simulink model "paralelo3usinas"  (Simulink 7.5)
settings: Solver=ode45  StartTime=0.0  StopTime=500  MaxStep=100  RelTol=1e-3
values from neighbouring files (symbols this model uses):
  B1 = 0.6    [princ_paralelo3usinas.m]
  B2 = 0.6    [princ_paralelo3usinas.m]
  C1 = 0.6    [princ_paralelo3usinas.m]
  C2 = 0.6    [princ_paralelo3usinas.m]
  DPD_pu1 = DPD/PB    (= 0.042296)    [sistema1.m]
  DPD_pu2 = DPD/PB    (= 0.070494)    [sistema2.m]
  DPD_pu3 = DPD/PB    (= 0.11279)    [sistema3.m]
  Gest = 0.0586    [princ_paralelo3usinas.m]
  Gsae = 0.1250    (= 0.125)    [princ_paralelo3usinas.m]
  K12 = cos(teta12)/X12    [princ_paralelo3usinas.m]
  K1_12 = sin (teta12)/X12    [princ_paralelo3usinas.m]
  K1_23 = sin (teta23)/X23    [princ_paralelo3usinas.m]
  K23 = cos(teta23)/X23    [princ_paralelo3usinas.m]
  K2_12 = sin(teta12)/X12    [princ_paralelo3usinas.m]
  Kd1 = 0.0586    [princ_paralelo3usinas.m]
  Kd2 = 3.2410    (= 3.241)    [princ_paralelo3usinas.m]
  Kd3 = 0.2826    [princ_paralelo3usinas.m]
  Ki1 = 0.0092    [princ_paralelo3usinas.m]
  Ki2 = 0.0541    [princ_paralelo3usinas.m]
  Kp1 = -0.0242    [princ_paralelo3usinas.m]
  Kp2 = -0.2928    [princ_paralelo3usinas.m]
  Kp3 = 0.3558    [princ_paralelo3usinas.m]
  Kps1 = 1/D_pu    (= 88.922039025)    [sistema1.m]
  Kps2 = 1/D_pu    (= 10.0350855099)    [sistema2.m]
  Kps3 = 1/D_pu    (= 15.8041808295)    [sistema3.m]
  PD_pu1 = PD/PB    (= 1.13594)    [sistema1.m]
  PD_pu2 = PD/PB    (= 1.893234)    [sistema2.m]
  REG_pu1 = REG/PB    (= 1.64172103535)    [sistema1.m]
  REG_pu2 = REG/PB    (= 1.31995425045)    [sistema2.m]
  REG_pu3 = REG/PB    (= 0.108094752772)    [sistema3.m]
  T1 = 0.1013    [princ_paralelo3usinas.m]
  T2 = 0.1238    [princ_paralelo3usinas.m]
  Ta = 0.4401    [princ_paralelo3usinas.m]
  Tb = 0.08    [princ_paralelo3usinas.m]
  Test = 0.0223    [princ_paralelo3usinas.m]
  TG1 = 0.6419    [sistema1.m]
  TG2 = 0.6002    [sistema2.m]
  TG3 = 0.4505    [sistema3.m]
  Tps1 = 2*H_pu/(D_pu*f0)    (= 48.2838817126)    [sistema1.m]
  Tps2 = 2*H_pu/(D_pu*f0)    (= 8.70581433357)    [sistema2.m]
  Tps3 = 2*H_pu/(D_pu*f0)    (= 1.06634811782)    [sistema3.m]
  Tt1 = 5.7257    [princ_paralelo3usinas.m]
  Tt2 = 1.0740    (= 1.074)    [princ_paralelo3usinas.m]
  Tt3 = 1.0552    [princ_paralelo3usinas.m]
  TW1 = 1.0882    [sistema1.m]
  TW2 = 1.2650    (= 1.265)    [sistema2.m]
  TW3 = 1.3430    (= 1.343)    [sistema3.m]
settings Model: Creator=Edimar  LastModifiedBy=Laís  ExtModeTrigMode=oneshot  ExtModeArmWhenConnect=off
settings DataIOCC: LimitDataPoints=off
settings OptimizationCC: BooleanDataType=off
settings DebuggingCC: SaveWithParameterizedLinksMsg=none  SignalResolutionControl=TryResolveAllWithWarning  SolverPrmCheckMsg=none  MultiTaskDSMMsg=warning  MultiTaskCondExecSysMsg=none  StrictBusMsg=None
settings HardwareCC: TargetUnknown=on
settings RTWCC: IncludeERTFirstTime=on

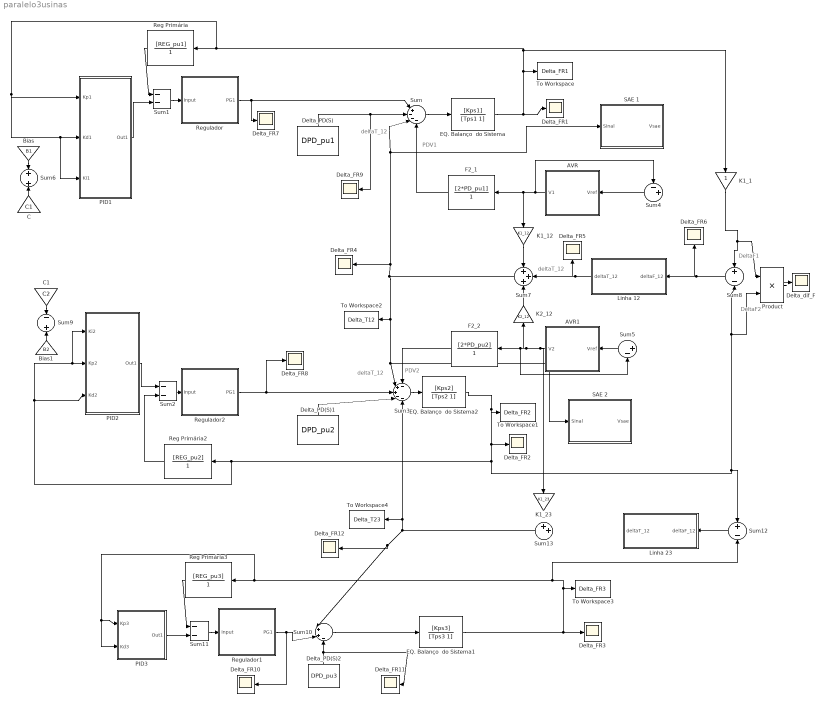
== system paralelo3usinas ==
  note: PDV1
  note: PDV2
  note: DeltaF1
  note: DeltaF2
  note: deltaT_12
  note: deltaT_12
  note: deltaT_12
  AVR : Subsystem
  AVR1 : Subsystem
  Bias : Gain  Gain=B1  ParameterDataType=fixdt(1, 16)  ParameterScaling=2^0  OutDataType=fixdt(1, 16)  OutScaling=2^0
  Bias1 : Gain  Gain=B2  ParameterDataType=fixdt(1, 16)  ParameterScaling=2^0  OutDataType=fixdt(1, 16)  OutScaling=2^0
  C : Gain  Gain=C1  ParameterDataType=fixdt(1, 16)  ParameterScaling=2^0  OutDataType=fixdt(1, 16)  OutScaling=2^0
  C1 : Gain  Gain=C2  ParameterDataType=fixdt(1, 16)  ParameterScaling=2^0  OutDataType=fixdt(1, 16)  OutScaling=2^0
  Delta_FR{1..12} (12 alike) : Scope
      Delta_FR1 settings: Description=tetetet  TimeRange=1000  YMin=-4  YMax=3
      Delta_FR10 settings: Description=tetetet  TimeRange=1000  YMin=-4  YMax=3  SaveName=ScopeData11  MaxDataPoints=5000000
      Delta_FR11 settings: Description=tetetet  TimeRange=1000  YMin=-4  YMax=3  SaveName=ScopeData12  MaxDataPoints=5000000
      Delta_FR12 settings: Description=tetetet  TimeRange=1000  YMin=-4  YMax=3  SaveName=ScopeData13  MaxDataPoints=5000000
      Delta_FR2 settings: Description=tetetet  TimeRange=1000  YMin=-4  YMax=3  SaveName=ScopeData3
      Delta_FR3 settings: Description=tetetet  TimeRange=1000  YMin=-4  YMax=3  SaveName=ScopeData9
      Delta_FR4 settings: Description=tetetet  TimeRange=1000  YMin=-4  YMax=3  SaveName=ScopeData8  MaxDataPoints=5000000
      Delta_FR5 settings: Description=tetetet  TimeRange=1000  YMin=-4  YMax=3  SaveName=ScopeData4
      Delta_FR6 settings: Description=tetetet  TimeRange=1000  YMin=-4  YMax=3  SaveName=ScopeData5
      Delta_FR7 settings: Description=tetetet  TimeRange=1000  YMin=-4  YMax=3  SaveName=ScopeData6  MaxDataPoints=5000000
      Delta_FR8 settings: Description=tetetet  TimeRange=1000  YMin=-4  YMax=3  SaveName=ScopeData7
      Delta_FR9 settings: Description=tetetet  TimeRange=1000  YMin=-4  YMax=3  SaveName=ScopeData10  MaxDataPoints=5000000
  Delta_PD(S) : Constant  Value=DPD_pu1
  Delta_PD(S)1 : Constant  Value=DPD_pu2
  Delta_PD(S)2 : Constant  Value=DPD_pu3
  Delta_dif_F : Scope
      settings: Description=tetetet  TimeRange=1000  YMin=-4  YMax=3
  EQ. Balanço  do Sistema : TransferFcn  Numerator=[Kps1]  Denominator=[Tps1 1]
  EQ. Balanço  do Sistema1 : TransferFcn  Numerator=[Kps3]  Denominator=[Tps3 1]
  EQ. Balanço  do Sistema2 : TransferFcn  Numerator=[Kps2]  Denominator=[Tps2 1]
  F2_1 : TransferFcn  Numerator=[2*PD_pu1]  Denominator=[0 1]
  F2_2 : TransferFcn  Numerator=[2*PD_pu2]  Denominator=[0 1]
  K1_1 : Gain  ParameterDataType=fixdt(1, 16)  ParameterScaling=2^0  OutDataType=fixdt(1, 16)  OutScaling=2^0
  K1_12 : Gain  Gain=K1_12  ParameterDataType=fixdt(1, 16)  ParameterScaling=2^0  OutDataType=fixdt(1, 16)  OutScaling=2^0
  K1_23 : Gain  Gain=K1_23  ParameterDataType=fixdt(1, 16)  ParameterScaling=2^0  OutDataType=fixdt(1, 16)  OutScaling=2^0
  K2_12 : Gain  Gain=K2_12  ParameterDataType=fixdt(1, 16)  ParameterScaling=2^0  OutDataType=fixdt(1, 16)  OutScaling=2^0
  Linha 12 : Subsystem
  Linha 23 : Subsystem
  PID1 : Subsystem
  PID2 : Subsystem
  PID3 : Subsystem
  Product : Product  OutDataType=fixdt(1, 16)  OutScaling=2^0  RndMeth=Zero
  Reg Primária : TransferFcn  Numerator=[REG_pu1]  Denominator=[0 1]
  Reg Primária2 : TransferFcn  Numerator=[REG_pu2]  Denominator=[0 1]
  Reg Primária3 : TransferFcn  Numerator=[REG_pu3]  Denominator=[0 1]
  Regulador : Subsystem
  Regulador1 : Subsystem
  Regulador2 : Subsystem
  SAE 1 : Subsystem
  SAE 2 : Subsystem
  Sum : Sum  Inputs=|+---  SaturateOnIntegerOverflow=on  InputSameDT=on  OutDataTypeStr=Inherit: Same as first input
  Sum1 : Sum  Inputs=--  SaturateOnIntegerOverflow=on  InputSameDT=on  OutDataTypeStr=Inherit: Same as first input
  Sum10 : Sum  Inputs=|++-  SaturateOnIntegerOverflow=on  InputSameDT=on  OutDataTypeStr=Inherit: Same as first input
  Sum11 : Sum  Inputs=--  SaturateOnIntegerOverflow=on  InputSameDT=on  OutDataTypeStr=Inherit: Same as first input
  Sum12 : Sum  Inputs=+|-  OutDataType=fixdt(1, 16)  OutScaling=2^0
  Sum13 : Sum  Inputs=++|  SaturateOnIntegerOverflow=on  InputSameDT=on  OutDataTypeStr=Inherit: Same as first input
  Sum2 : Sum  Inputs=--  SaturateOnIntegerOverflow=on  InputSameDT=on  OutDataTypeStr=Inherit: Same as first input
  Sum3 : Sum  Inputs=-++--  SaturateOnIntegerOverflow=on  InputSameDT=on  OutDataTypeStr=Inherit: Same as first input
  Sum4 : Sum  Inputs=-+|  SaturateOnIntegerOverflow=on  InputSameDT=on  OutDataTypeStr=Inherit: Same as first input
  Sum5 : Sum  Inputs=|+-  SaturateOnIntegerOverflow=on  InputSameDT=on  OutDataTypeStr=Inherit: Same as first input
  Sum6 : Sum  Inputs=+|+  SaturateOnIntegerOverflow=on  InputSameDT=on  OutDataTypeStr=Inherit: Same as first input
  Sum7 : Sum  Inputs=+++  SaturateOnIntegerOverflow=on  InputSameDT=on  OutDataTypeStr=Inherit: Same as first input
  Sum8 : Sum  Inputs=+|-  OutDataType=fixdt(1, 16)  OutScaling=2^0
  Sum9 : Sum  Inputs=-|+  SaturateOnIntegerOverflow=on  InputSameDT=on  OutDataTypeStr=Inherit: Same as first input
  To Workspace : ToWorkspace  VariableName=Delta_FR1  SampleTime=-1  SaveFormat=Array
  To Workspace1 : ToWorkspace  VariableName=Delta_FR2  SampleTime=-1  SaveFormat=Array
  To Workspace2 : ToWorkspace  VariableName=Delta_T12  SampleTime=-1  SaveFormat=Array
  To Workspace3 : ToWorkspace  VariableName=Delta_FR3  SampleTime=-1  SaveFormat=Array
  To Workspace4 : ToWorkspace  VariableName=Delta_T23  SampleTime=-1  SaveFormat=Array
  wires:
  Delta_PD(S)/1 -> Sum/2, Delta_FR9/1
  EQ. Balanço  do Sistema/1 -> Delta_FR1/1, To Workspace/1, Reg Primária/1, PID1/1(Kp1), PID1/2(Kd1), PID1/3(Ki1), K1_1/1
  Sum/1 -> EQ. Balanço  do Sistema/1
  AVR/1(V1) -> Sum4/1, F2_1/1, K1_12/1
  Sum4/1 -> AVR/1(Vref)
  Sum3/1 -> EQ. Balanço  do Sistema2/1
  EQ. Balanço  do Sistema2/1 -> To Workspace1/1, Delta_FR2/1, Reg Primária2/1, PID2/3(Kd2), PID2/2(Kp2), PID2/1(Ki2), Product/2, Sum8/2, Sum12/1
  Sum5/1 -> AVR1/1(Vref)
  AVR1/1(V2) -> Sum5/2, F2_2/1, K2_12/1, K1_23/1
  F2_2/1 -> Sum3/1
  Delta_PD(S)1/1 -> Sum3/4
  F2_1/1 -> Sum/4
  PID1/1(Out1) -> Sum1/2
  Reg Primária/1 -> Sum1/1
  Sum1/1 -> Regulador/1(Input)
  Regulador/1(PG1) -> Sum/1, Delta_FR7/1
  Sum2/1 -> Regulador2/1(Input)
  PID2/1(Out1) -> Sum2/1
  Reg Primária2/1 -> Sum2/2
  Regulador2/1(PG1) -> Sum3/3, Delta_FR8/1
  Linha 12/1(deltaT_12) -> Sum7/2, Delta_FR5/1
  Product/1 -> Delta_dif_F/1
  Sum8/1 -> Linha 12/1(deltaF_12), Delta_FR6/1
  K1_1/1 -> Product/1, Sum8/1
  Sum7/1 -> Delta_FR4/1, Sum/3, SAE 1/1(Sinal), To Workspace2/1, Sum3/2, SAE 2/1(Sinal)
  K2_12/1 -> Sum7/3
  K1_12/1 -> Sum7/1
  Bias/1 -> Sum6/1
  C/1 -> Sum6/2
  C1/1 -> Sum9/1
  Bias1/1 -> Sum9/2
  EQ. Balanço  do Sistema1/1 -> Delta_FR3/1, To Workspace3/1, Reg Primária3/1, PID3/1(Kp3), PID3/2(Kd3), Sum12/2
  Sum10/1 -> EQ. Balanço  do Sistema1/1
  PID3/1(Out1) -> Sum11/2
  Reg Primária3/1 -> Sum11/1
  Sum11/1 -> Regulador1/1(Input)
  Sum12/1 -> Linha 23/1(deltaF_12)
  Regulador1/1(PG1) -> Sum10/2, Delta_FR10/1
  Delta_PD(S)2/1 -> Sum10/3, Delta_FR11/1
  Sum13/1 -> Sum3/5, To Workspace4/1, Sum10/1, Delta_FR12/1

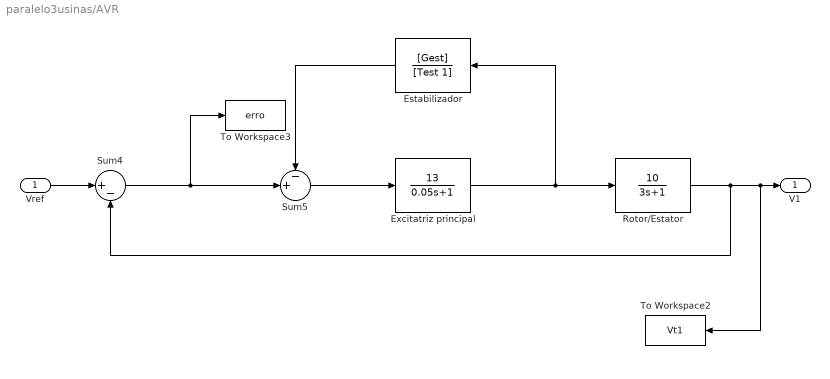
== system paralelo3usinas/AVR ==
  Vref : Inport
  Estabilizador : TransferFcn  Numerator=[Gest]  Denominator=[Test 1]
  Excitatriz principal : TransferFcn  Numerator=[13]  Denominator=[0.05 1]
  Rotor/Estator : TransferFcn  Numerator=[10]  Denominator=[3 1]
  Sum4 : Sum  Inputs=|+-  SaturateOnIntegerOverflow=on  InputSameDT=on  OutDataTypeStr=Inherit: Same as first input
  Sum5 : Sum  Inputs=-+|  SaturateOnIntegerOverflow=on  InputSameDT=on  OutDataTypeStr=Inherit: Same as first input
  To Workspace2 : ToWorkspace  VariableName=Vt1  SampleTime=-1  SaveFormat=Array
  To Workspace3 : ToWorkspace  VariableName=erro  SampleTime=-1  SaveFormat=Array
  V1 : Outport
  wires:
  Excitatriz principal/1 -> Rotor/Estator/1, Estabilizador/1
  Estabilizador/1 -> Sum5/1
  Sum4/1 -> Sum5/2, To Workspace3/1
  Sum5/1 -> Excitatriz principal/1
  Rotor/Estator/1 -> To Workspace2/1, V1/1, Sum4/2
  Vref/1 -> Sum4/1

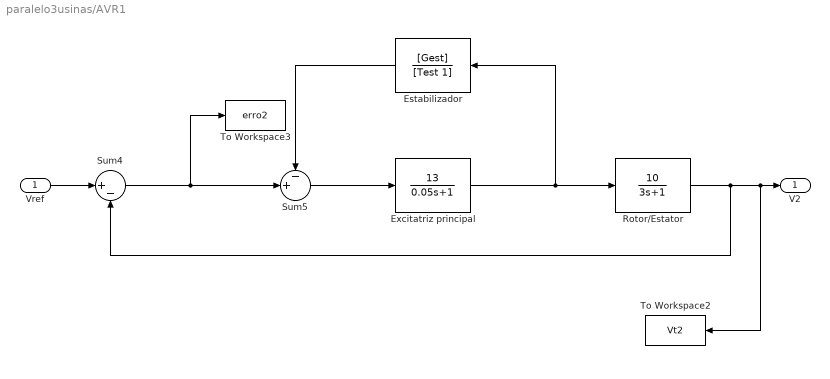
== system paralelo3usinas/AVR1 ==
  Vref : Inport
  Estabilizador : TransferFcn  Numerator=[Gest]  Denominator=[Test 1]
  Excitatriz principal : TransferFcn  Numerator=[13]  Denominator=[0.05 1]
  Rotor/Estator : TransferFcn  Numerator=[10]  Denominator=[3 1]
  Sum4 : Sum  Inputs=|+-  SaturateOnIntegerOverflow=on  InputSameDT=on  OutDataTypeStr=Inherit: Same as first input
  Sum5 : Sum  Inputs=-+|  SaturateOnIntegerOverflow=on  InputSameDT=on  OutDataTypeStr=Inherit: Same as first input
  To Workspace2 : ToWorkspace  VariableName=Vt2  SampleTime=-1  SaveFormat=Array
  To Workspace3 : ToWorkspace  VariableName=erro2  SampleTime=-1  SaveFormat=Array
  V2 : Outport
  wires:
  Excitatriz principal/1 -> Rotor/Estator/1, Estabilizador/1
  Estabilizador/1 -> Sum5/1
  Sum4/1 -> Sum5/2, To Workspace3/1
  Sum5/1 -> Excitatriz principal/1
  Rotor/Estator/1 -> To Workspace2/1, V2/1, Sum4/2
  Vref/1 -> Sum4/1

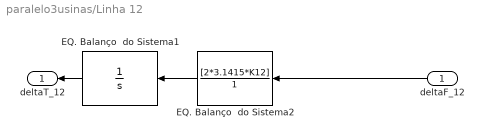
== system paralelo3usinas/Linha 12 ==
  deltaF_12 : Inport
  EQ. Balanço  do Sistema1 : TransferFcn  Denominator=[1 0]
  EQ. Balanço  do Sistema2 : TransferFcn  Numerator=[2*3.1415*K12]  Denominator=[1]
  deltaT_12 : Outport
  wires:
  EQ. Balanço  do Sistema2/1 -> EQ. Balanço  do Sistema1/1
  EQ. Balanço  do Sistema1/1 -> deltaT_12/1
  deltaF_12/1 -> EQ. Balanço  do Sistema2/1

== system paralelo3usinas/Linha 23 ==
  deltaF_12 : Inport
  EQ. Balanço  do Sistema1 : TransferFcn  Denominator=[1 0]
  EQ. Balanço  do Sistema2 : TransferFcn  Numerator=[2*3.1415*K23]  Denominator=[1]
  deltaT_12 : Outport
  wires:
  EQ. Balanço  do Sistema2/1 -> EQ. Balanço  do Sistema1/1
  EQ. Balanço  do Sistema1/1 -> deltaT_12/1
  deltaF_12/1 -> EQ. Balanço  do Sistema2/1

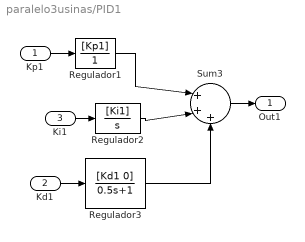
== system paralelo3usinas/PID1 ==
  Kp1 : Inport
  Kd1 : Inport  Port=2
  Ki1 : Inport  Port=3
  Regulador1 : TransferFcn  Numerator=[Kp1]  Denominator=[1]
  Regulador2 : TransferFcn  Numerator=[Ki1]  Denominator=[1 0]
  Regulador3 : TransferFcn  Numerator=[Kd1 0]  Denominator=[0.5 1]
  Sum3 : Sum  Inputs=|+++  OutDataType=fixdt(1, 16)  OutScaling=2^0
  Out1 : Outport
  wires:
  Regulador1/1 -> Sum3/1
  Regulador2/1 -> Sum3/2
  Regulador3/1 -> Sum3/3
  Kp1/1 -> Regulador1/1
  Sum3/1 -> Out1/1
  Ki1/1 -> Regulador2/1
  Kd1/1 -> Regulador3/1

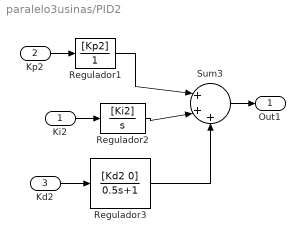
== system paralelo3usinas/PID2 ==
  Ki2 : Inport
  Kp2 : Inport  Port=2
  Kd2 : Inport  Port=3
  Regulador1 : TransferFcn  Numerator=[Kp2]  Denominator=[1]
  Regulador2 : TransferFcn  Numerator=[Ki2]  Denominator=[1 0]
  Regulador3 : TransferFcn  Numerator=[Kd2 0]  Denominator=[0.5 1]
  Sum3 : Sum  Inputs=|+++  OutDataType=fixdt(1, 16)  OutScaling=2^0
  Out1 : Outport
  wires:
  Regulador1/1 -> Sum3/1
  Regulador2/1 -> Sum3/2
  Regulador3/1 -> Sum3/3
  Kp2/1 -> Regulador1/1
  Sum3/1 -> Out1/1
  Ki2/1 -> Regulador2/1
  Kd2/1 -> Regulador3/1

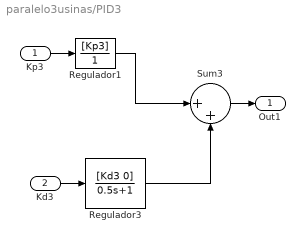
== system paralelo3usinas/PID3 ==
  Kp3 : Inport
  Kd3 : Inport  Port=2
  Regulador1 : TransferFcn  Numerator=[Kp3]  Denominator=[1]
  Regulador3 : TransferFcn  Numerator=[Kd3 0]  Denominator=[0.5 1]
  Sum3 : Sum  Inputs=|++  OutDataType=fixdt(1, 16)  OutScaling=2^0
  Out1 : Outport
  wires:
  Regulador1/1 -> Sum3/1
  Kp3/1 -> Regulador1/1
  Sum3/1 -> Out1/1
  Kd3/1 -> Regulador3/1
  Regulador3/1 -> Sum3/2

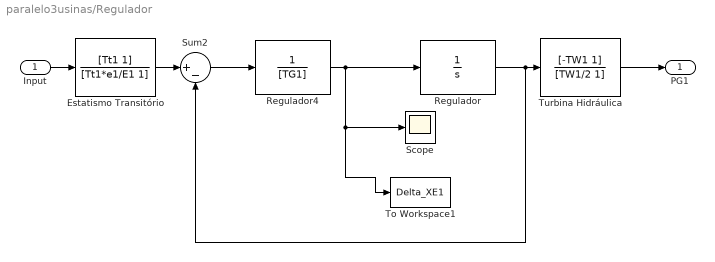
== system paralelo3usinas/Regulador ==
  Input : Inport
  Estatismo Transitório : TransferFcn  Numerator=[Tt1 1]  Denominator=[Tt1*e1/E1 1]
  Regulador : TransferFcn  Denominator=[1 0]
  Regulador4 : TransferFcn  Denominator=[TG1]
  Scope : Scope
      settings: SaveName=ScopeData2
  Sum2 : Sum  Inputs=|+-  SaturateOnIntegerOverflow=on  InputSameDT=on  OutDataTypeStr=Inherit: Same as first input
  To Workspace1 : ToWorkspace  VariableName=Delta_XE1  SampleTime=-1  SaveFormat=Array
  Turbina Hidráulica : TransferFcn  Numerator=[-TW1 1]  Denominator=[TW1/2 1]
  PG1 : Outport
  wires:
  Turbina Hidráulica/1 -> PG1/1
  Regulador/1 -> Turbina Hidráulica/1, Sum2/2
  Regulador4/1 -> Regulador/1, To Workspace1/1, Scope/1
  Estatismo Transitório/1 -> Sum2/1
  Sum2/1 -> Regulador4/1
  Input/1 -> Estatismo Transitório/1

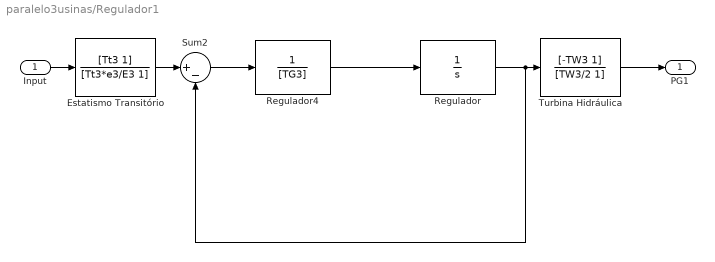
== system paralelo3usinas/Regulador1 ==
  Input : Inport
  Estatismo Transitório : TransferFcn  Numerator=[Tt3 1]  Denominator=[Tt3*e3/E3 1]
  Regulador : TransferFcn  Denominator=[1 0]
  Regulador4 : TransferFcn  Denominator=[TG3]
  Sum2 : Sum  Inputs=|+-  SaturateOnIntegerOverflow=on  InputSameDT=on  OutDataTypeStr=Inherit: Same as first input
  Turbina Hidráulica : TransferFcn  Numerator=[-TW3 1]  Denominator=[TW3/2 1]
  PG1 : Outport
  wires:
  Turbina Hidráulica/1 -> PG1/1
  Regulador/1 -> Turbina Hidráulica/1, Sum2/2
  Regulador4/1 -> Regulador/1
  Estatismo Transitório/1 -> Sum2/1
  Sum2/1 -> Regulador4/1
  Input/1 -> Estatismo Transitório/1

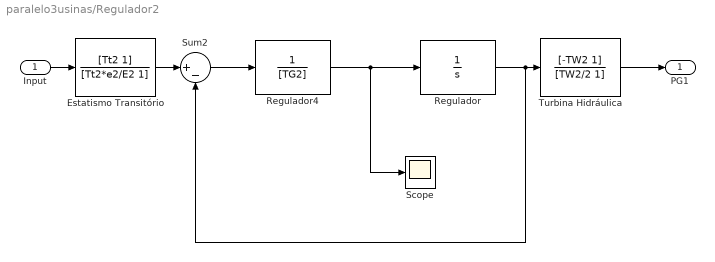
== system paralelo3usinas/Regulador2 ==
  Input : Inport
  Estatismo Transitório : TransferFcn  Numerator=[Tt2 1]  Denominator=[Tt2*e2/E2 1]
  Regulador : TransferFcn  Denominator=[1 0]
  Regulador4 : TransferFcn  Denominator=[TG2]
  Scope : Scope
      settings: SaveName=ScopeData2
  Sum2 : Sum  Inputs=|+-  SaturateOnIntegerOverflow=on  InputSameDT=on  OutDataTypeStr=Inherit: Same as first input
  Turbina Hidráulica : TransferFcn  Numerator=[-TW2 1]  Denominator=[TW2/2 1]
  PG1 : Outport
  wires:
  Turbina Hidráulica/1 -> PG1/1
  Regulador/1 -> Turbina Hidráulica/1, Sum2/2
  Regulador4/1 -> Regulador/1, Scope/1
  Estatismo Transitório/1 -> Sum2/1
  Sum2/1 -> Regulador4/1
  Input/1 -> Estatismo Transitório/1

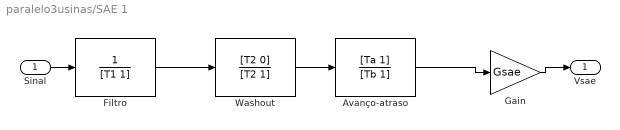
== system paralelo3usinas/SAE 1 ==
  Sinal : Inport
  Avanço-atraso : TransferFcn  Numerator=[Ta 1]  Denominator=[Tb 1]
  Filtro : TransferFcn  Denominator=[T1 1]
  Gain : Gain  Gain=Gsae  ParameterDataType=fixdt(1, 16)  ParameterScaling=2^0  OutDataType=fixdt(1, 16)  OutScaling=2^0
  Washout : TransferFcn  Numerator=[T2 0]  Denominator=[T2 1]
  Vsae : Outport
  wires:
  Filtro/1 -> Washout/1
  Washout/1 -> Avanço-atraso/1
  Sinal/1 -> Filtro/1
  Gain/1 -> Vsae/1
  Avanço-atraso/1 -> Gain/1

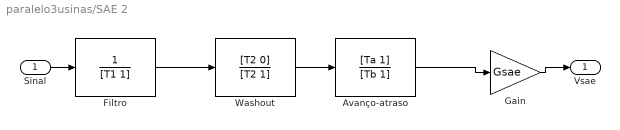
== system paralelo3usinas/SAE 2 ==
  Sinal : Inport
  Avanço-atraso : TransferFcn  Numerator=[Ta 1]  Denominator=[Tb 1]
  Filtro : TransferFcn  Denominator=[T1 1]
  Gain : Gain  Gain=Gsae  ParameterDataType=fixdt(1, 16)  ParameterScaling=2^0  OutDataType=fixdt(1, 16)  OutScaling=2^0
  Washout : TransferFcn  Numerator=[T2 0]  Denominator=[T2 1]
  Vsae : Outport
  wires:
  Filtro/1 -> Washout/1
  Washout/1 -> Avanço-atraso/1
  Sinal/1 -> Filtro/1
  Gain/1 -> Vsae/1
  Avanço-atraso/1 -> Gain/1
